simulink model "PhiTheta"  (R2014a)
settings: Solver=ode45  StartTime=0.0  StopTime=15  RelTol=1e-3
values from neighbouring files (symbols this model uses):
  satThrust = 10000    [decoupled.m]
undefined symbols (not defined in the file or in its folder): den_tf_cont, num_tf_cont, sigbuilder_block
settings Model: Creator=userk  LastModifiedBy=root
settings DataIOCC: SignalLoggingSaveFormat=ModelDataLogs
settings OptimizationCC: ExpressionDepthLimit=2147483647
settings DebuggingCC: UnderspecifiedInitializationDetection=Classic  FcnCallInpInsideContextMsg=EnableAllAsWarning  StateNameClashWarn=warning

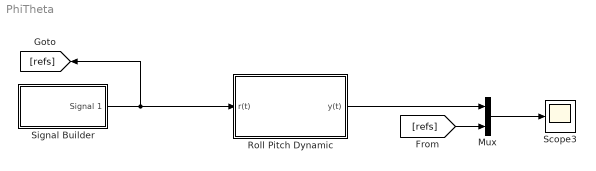
== system PhiTheta ==
  Mux : Mux  Inputs=2
  Roll Pitch Dynamic : Subsystem
  Scope3 : Scope
  Signal Builder : Subsystem  Tag=STV Subsys  LoadFcn=sigbuilder_block('load');  StartFcn=sigbuilder_block('start');  StopFcn=sigbuilder_block('stop');  ClipboardFcn=sigbuilder_block('clipboard');  mask(Sigbuilder block){}
      mask help: Simulink:masks:SigbuilderBlock_MD
      mask init:
      | if ~strcmp(get_param(bdroot(gcbh),'SimulationStatus'),'stopped') tuvar = sigbuilder_block('maskInit'); end
      settings: CopyFcn=sigbuilder_block('copy');  DeleteFcn=sigbuilder_block('delete');  ModelCloseFcn=sigbuilder_block('modelClose');  PreSaveFcn=sigbuilder_block('preSave');  PauseFcn=sigbuilder_block('pause');  ContinueFcn=sigbuilder_block('continue');  NameChangeFcn=sigbuilder_block('namechange');  OpenFcn=sigbuilder_block('open',[265.6 120.8 550.4 400 ]);  CloseFcn=sigbuilder_block('close');
      mask Display: plot(0, 0, 100, 100,[2, 2, 32, 32, 2], [68, 8, 8, 68, 68],[32, 2], [38, 38], [32, 19, 2],[53, 60, 44], [32, 17, 17, 2],[16, 16, 31, 31]);txt = getActiveGroup(gcbh);text(2, 100, txt,'verticalAlignment', 'top');
  wires:
  Signal Builder/1(Signal 1) -> [refs], Roll Pitch Dynamic/1(r(t))
  [refs] -> Mux/2
  Mux/1 -> Scope3/1
  Roll Pitch Dynamic/1(y(t)) -> Mux/1

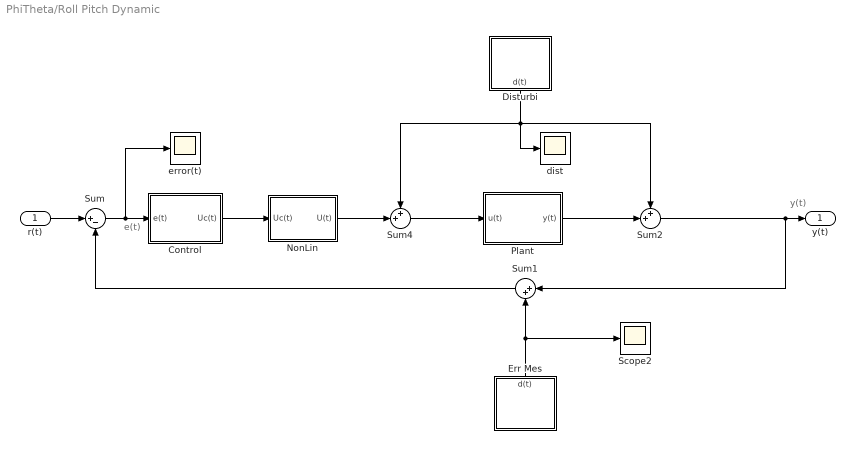
== system PhiTheta/Roll Pitch Dynamic ==
  note: e(t)
  note: y(t)
  r(t) : Inport
  Control : Subsystem
  Disturbi : Subsystem
  Err Mes : Subsystem
  NonLin : Subsystem
  Plant : Subsystem
  Scope2 : Scope
      settings: SaveName=ScopeData2
  Sum : Sum  Inputs=|+-
  Sum1 : Sum  Inputs=|++
  Sum2 : Sum  Inputs=++|
  Sum4 : Sum  Inputs=++|
  dist : Scope
  error(t) : Scope
      settings: SaveName=ScopeData4
  y(t) : Outport
  wires:
  Sum/1 -> error(t)/1, Control/1(e(t))
  Plant/1(y(t)) -> Sum2/2
  Sum2/1 -> Sum1/1, y(t)/1
  Sum1/1 -> Sum/2
  Disturbi/1("  d(t)") -> dist/1, Sum4/1, Sum2/1
  Sum4/1 -> Plant/1(u(t))
  Control/1(Uc(t)) -> NonLin/1(Uc(t))
  NonLin/1(U(t)) -> Sum4/2
  r(t)/1 -> Sum/1
  Err Mes/1("  d(t)") -> Sum1/2, Scope2/1

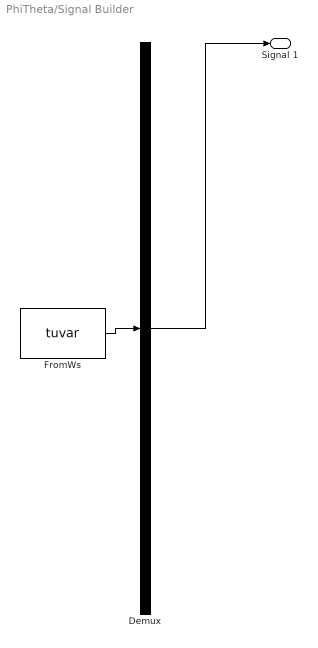
== system PhiTheta/Signal Builder ==
  Demux : Demux  Tag=STV Demux  Outputs=1
  FromWs : FromWorkspace  Tag=STV FromWs  VariableName=tuvar  SampleTime=0
      SigBuilderData=|
      | common.afterFinalStr = 'Extrapolate'
      | common.sampleTime = 0
      | dataSet.timeRange = [0 10]
      | dataSet.name = 'Group 1'
      | sbobj.Groups.Name = 'Group 1'
      | sbobj.Groups.Signals.Name = 'Signal 1'
      | sbobj.Groups.Signals.XData = [0 4.06 4.06 6 6 10]
      | sbobj.Groups.Signals.YData = [-0.005 0.05 1 1 0.995 0.01]
  Signal 1 : Outport  Tag=STV Outport
  wires:
  Demux/1 -> Signal 1/1
  FromWs/1 -> Demux/1

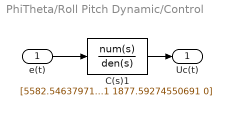
== system PhiTheta/Roll Pitch Dynamic/Control ==
  e(t) : Inport
  C(s)1 : TransferFcn  Numerator=[5582.54637971166 77190.9890523944 0]  Denominator=[1 1877.59274550691 0]
  Uc(t) : Outport
  wires:
  e(t)/1 -> C(s)1/1
  C(s)1/1 -> Uc(t)/1

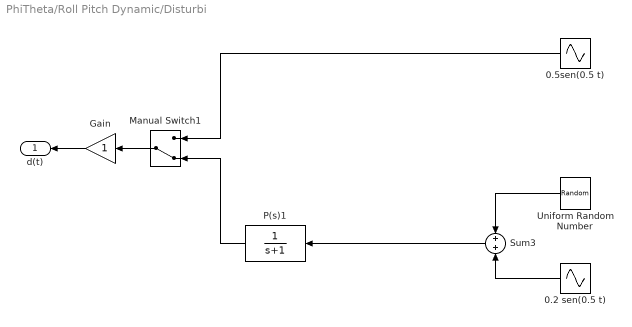
== system PhiTheta/Roll Pitch Dynamic/Disturbi ==
  0.2 sen(0.5 t) : Sin  Amplitude=0.2  Frequency=0.4  Phase=1  SampleTime=0
  0.5sen(0.5 t) : Sin  Amplitude=0.5  Frequency=0.5  Phase=1  SampleTime=0
  Gain : Gain
  Manual Switch1 : ManualSwitch  CurrentSetting=0
  P(s)1 : TransferFcn  Numerator=1  Denominator=[1 1]
  Sum3 : Sum
  Uniform Random Number : UniformRandomNumber  Minimum=-0.5  Maximum=0.5  SampleTime=0.1
  "  d(t)" : Outport
  wires:
  Uniform Random Number/1 -> Sum3/1
  0.2 sen(0.5 t)/1 -> Sum3/2
  Sum3/1 -> P(s)1/1
  0.5sen(0.5 t)/1 -> Manual Switch1/1
  P(s)1/1 -> Manual Switch1/2
  Gain/1 -> "  d(t)"/1
  Manual Switch1/1 -> Gain/1

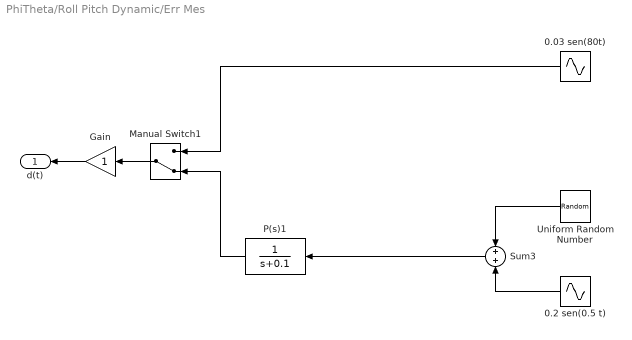
== system PhiTheta/Roll Pitch Dynamic/Err Mes ==
  0.03 sen(80t) : Sin  Amplitude=0.003  Frequency=80  Phase=1  SampleTime=0
  0.2 sen(0.5 t) : Sin  Amplitude=0.02  Frequency=50  Phase=1  SampleTime=0
  Gain : Gain
  Manual Switch1 : ManualSwitch  CurrentSetting=0
  P(s)1 : TransferFcn  Numerator=1  Denominator=[1 0.1]
  Sum3 : Sum
  Uniform Random Number : UniformRandomNumber  Minimum=-0.05  Maximum=0.05  SampleTime=0.1
  "  d(t)" : Outport
  wires:
  Uniform Random Number/1 -> Sum3/1
  0.2 sen(0.5 t)/1 -> Sum3/2
  Sum3/1 -> P(s)1/1
  0.03 sen(80t)/1 -> Manual Switch1/1
  P(s)1/1 -> Manual Switch1/2
  Gain/1 -> "  d(t)"/1
  Manual Switch1/1 -> Gain/1

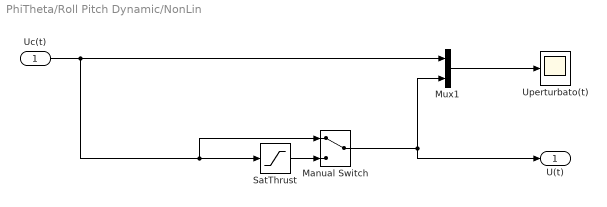
== system PhiTheta/Roll Pitch Dynamic/NonLin ==
  Uc(t) : Inport
  Manual Switch : ManualSwitch
  Mux1 : Mux  Inputs=2
  SatThrust : Saturate  UpperLimit=satThrust  LowerLimit=-6
  Uperturbato(t) : Scope
      settings: ShowLegends=on  TimeRange=15  YMin=-150000  YMax=250000  SaveName=ScopeData5
  U(t) : Outport
  wires:
  Uc(t)/1 -> Mux1/1, Manual Switch/1, SatThrust/1
  Mux1/1 -> Uperturbato(t)/1
  SatThrust/1 -> Manual Switch/2
  Manual Switch/1 -> U(t)/1, Mux1/2

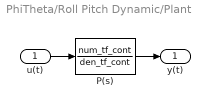
== system PhiTheta/Roll Pitch Dynamic/Plant ==
  u(t) : Inport
  P(s) : TransferFcn  Numerator=num_tf_cont  Denominator=den_tf_cont
  y(t) : Outport
  wires:
  u(t)/1 -> P(s)/1
  P(s)/1 -> y(t)/1
